simulink model "hw2_q5"  (R2022b)
settings: Solver=ode4  StartTime=0.0  StopTime=10.0  FixedStep=0.001  RelTol=1e-3
settings Model: Creator=gaura  LastModifiedBy=gaura

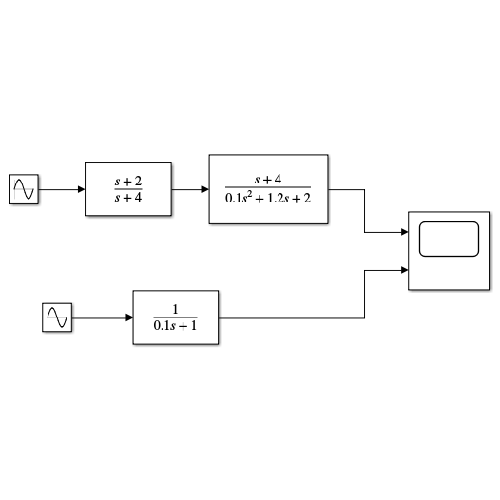
[thumbnail: Simulink's stored preview of the top-level diagram]
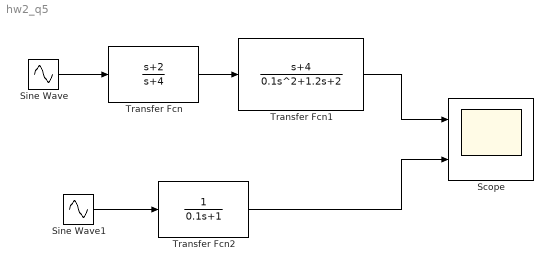
== system hw2_q5 ==
  Scope : Scope  NumInputPorts=2
  Sine Wave : Sin  Frequency=2  SampleTime=0
  Sine Wave1 : Sin  Frequency=2  SampleTime=0
  Transfer Fcn : TransferFcn  Numerator=[1 2]  Denominator=[1 4]
  Transfer Fcn1 : TransferFcn  Numerator=[1 4]  Denominator=[0.1 1.2 2]
  Transfer Fcn2 : TransferFcn  Denominator=[0.1 1]
  wires:
  Sine Wave/1 -> Transfer Fcn/1
  Transfer Fcn/1 -> Transfer Fcn1/1
  Transfer Fcn1/1 -> Scope/1
  Sine Wave1/1 -> Transfer Fcn2/1
  Transfer Fcn2/1 -> Scope/2
